simulink model "sim_state_space_DC"  (R2022b)
settings: Solver=ode5  StartTime=0.0  StopTime=t_s  FixedStep=h  RelTol=1e-3
undefined symbols (not defined in the file): A, B, C, Step
settings Model: Creator=Claudia  LastModifiedBy=Claudia Yasar
settings SolverCC: AlgebraicLoopSolver=TrustRegion
settings DataIOCC: ReturnWorkspaceOutputs=off
settings DebuggingCC: UnconnectedInputMsg=warning  UnconnectedOutputMsg=warning  UnconnectedLineMsg=warning  SFMachineParentedDataDiag=warning  ArithmeticOperatorsInVariantConditions=warning
settings ModelReferenceCC: EnableRefExpFcnMdlSchedulingChecks=on
settings SFSimCC: CustomCodeUndefinedFunction=UseInterfaceOnly
settings RTWCC: DLArmComputeVersion=19.05

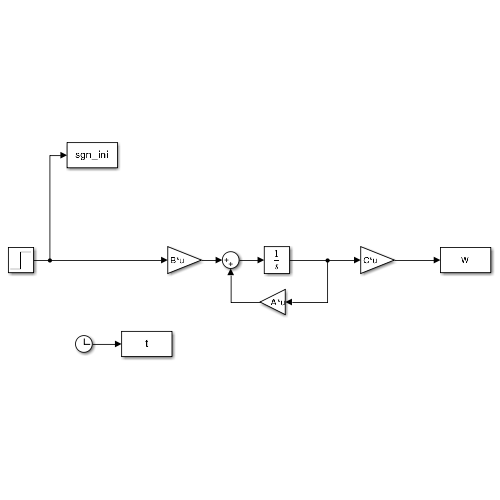
[thumbnail: Simulink's stored preview of the top-level diagram]
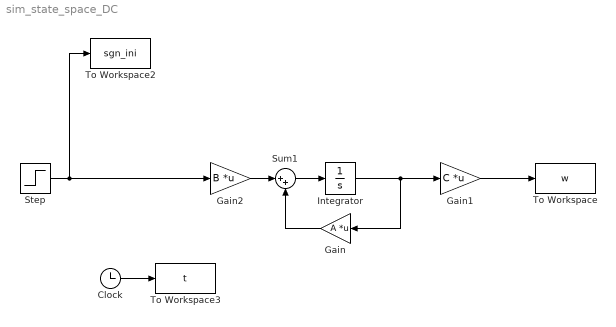
== system sim_state_space_DC ==
  Clock : Clock
  Gain : Gain  Gain=A  Multiplication=Matrix(K*u)
  Gain1 : Gain  Gain=C  Multiplication=Matrix(K*u)
  Gain2 : Gain  Gain=B  Multiplication=Matrix(K*u)
  Integrator : Integrator  IgnoreLimit=on
  Step : Step  Time=0  After=Step  SampleTime=0
  Sum1 : Sum  Inputs=|++
  To Workspace : ToWorkspace  VariableName=w  SampleTime=-1
  To Workspace2 : ToWorkspace  VariableName=sgn_ini  SampleTime=-1
      settings: OpenFcn=figure, plot(t,senal), xlabel('tiempo(s)'), ylabel('posicion')
  To Workspace3 : ToWorkspace  VariableName=t  SampleTime=-1
      settings: OpenFcn=figure, plot(t,entrada), xlabel('tiempo(s)'), ylabel('posicion')
  wires:
  Gain2/1 -> Sum1/1
  Sum1/1 -> Integrator/1
  Integrator/1 -> Gain/1, Gain1/1
  Gain1/1 -> To Workspace/1
  Gain/1 -> Sum1/2
  Clock/1 -> To Workspace3/1
  Step/1 -> Gain2/1, To Workspace2/1
